simulink model "MMC_model"  (R2024b)
settings: Solver=ode23t  StartTime=0.0  StopTime=0.5  RelTol=1e-3
undefined symbols (not defined in the file): C0, f0, fs, L, Larm, Ldc, Rarm, Rdc, Ts
libraries: spsHalfBridgeMMCLib x36, spsSeriesRLCBranchLib x10, eePwmGeneratorMultilevel x6, spsDCVoltageSourceLib x2, spsGroundLib x1, spsThreePhaseSeriesRLCLoadLib x1, spsThreePhaseVIMeasurementLib x1, sps_lib x1
settings Model: Creator=nana  LastModifiedBy=nana

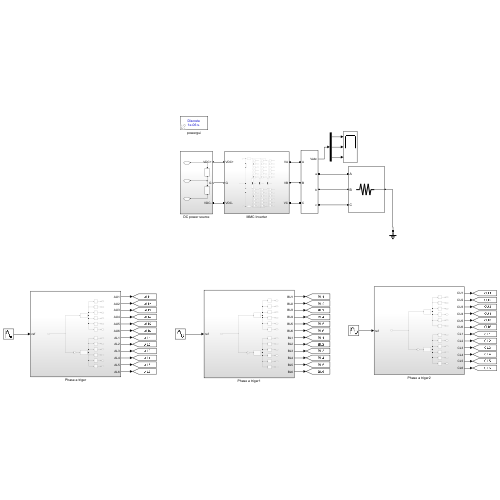
[thumbnail: Simulink's stored preview of the top-level diagram]
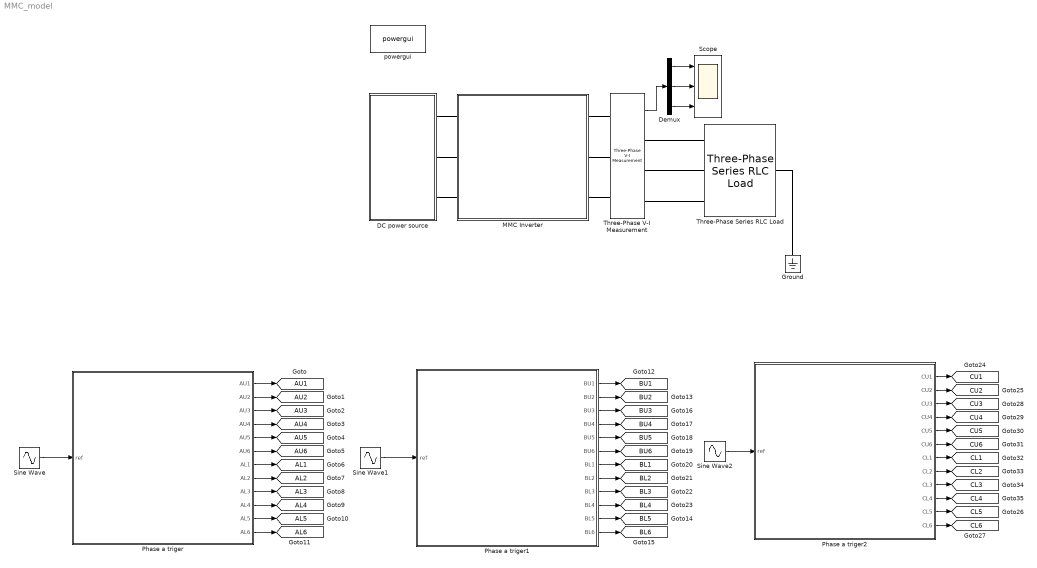
== system MMC_model ==
  DC power source : Subsystem
  Demux : Demux  Outputs=3
  Ground : spsGroundLib/Ground  LConnTagsString=a
  MMC Inverter : Subsystem
  Phase a triger : Subsystem
  Phase a triger1 : Subsystem
  Phase a triger2 : Subsystem
  Scope : Scope  NumInputPorts=3
  Sine Wave : Sin  Frequency=2*pi*f0  SampleTime=Ts
  Sine Wave1 : Sin  Frequency=2*pi*f0  Phase=-2*pi/3  SampleTime=Ts
  Sine Wave2 : Sin  Frequency=2*pi*f0  Phase=+2*pi/3  SampleTime=Ts
  Three-Phase Series RLC Load : spsThreePhaseSeriesRLCLoadLib/Three-Phase Series RLC Load  LConnTagsString=A|B|C  RConnTagsString=N  Configuration=Y (neutral)  NominalVoltage=12000  Vabc=[1e3 1e3 1e3]  Vabcp=[1e3 1e3 1e3]  NominalFrequency=50  UnbalancedPower=off  ActivePower=20e3  InductivePower=0  CapacitivePower=0  Pabc=[10e3 9e3 11e3]  QLabc=[100 90 110]  QCabc=[100 90 110]  Pabcp=[10e3 9e3 11e3]  QLabcp=[100 90 110]  QCabcp=[100 90 110]  Measurements=None  LoadType=constant Z
  Three-Phase V-I Measurement : spsThreePhaseVIMeasurementLib/Three-Phase V-I Measurement  VoltageMeasurement=phase-to-ground  SetLabelV=off  LabelV=Vabc  Vpu=off  VpuLL=off  CurrentMeasurement=yes  SetLabelI=on  LabelI=Iabc  Ipu=off  Pbase=100e6  Vbase=500e3  OutputType=Complex  PhasorSimulation=off  PSBequivalent=0
  powergui : sps_lib/powergui  Priority=1  SimulationMode=Discrete  SampleTime=1e-6  frequency=60  Iterations=50  frequencyindice=0  Pbase=100e6  ErrMax=1e-4  UnitsV=kV  UnitsW=MW  buscounter=0  FunctionMessages=off  echomessages=off  EnableUseOfTLC=off  CurrentSourceSwitches=off  DisableSnubberDevices=off  DisableRonSwitches=off  DisableVfSwitches=off  DisplayEquations=off  AutomaticDiscreteSolvers=off  SolverType=Tustin/Backward Euler (TBE)  Interpol=off  ExternalGateDelay=off  methode=off  Ts=100  x0status=blocks  SPID=on  SwTol=0  HookPort=off  NonlinearTolerance=1e-4  nMaxIteration=100  ContinueOnMaxIteration=off  RestoreLinks=warning  ResistiveCurrentMeasurement=off  Frange=[0:2:500]  Ylog=off  Xlog=on  ShowGrid=off  save=off  variable=ZData  structure=0  ZoomFFT=off  StartTime=0.0  cycles=1  DisplayStyle=1  fundamental=60  FreqAxis=off  MaxFrequency=1000  frequencyindicesteady=1  RmsSteady=1  display=off
  tag scope: AL1=global, AL2=global, AL3=global, AL4=global, AL5=global, AL6=global, AU1=global, AU2=global, AU3=global, AU4=global, AU5=global, AU6=global, BL1=global, BL2=global, BL3=global, BL4=global, BL5=global, BL6=global, BU1=global, BU2=global, BU3=global, BU4=global, BU5=global, BU6=global, CL1=global, CL2=global, CL3=global, CL4=global, CL5=global, CL6=global, CU1=global, CU2=global, CU3=global, CU4=global, CU5=global, CU6=global
  wires:
  Sine Wave/1 -> Phase a triger/1(ref)
  Sine Wave1/1 -> Phase a triger1/1(ref)
  Sine Wave2/1 -> Phase a triger2/1(ref)
  Phase a triger/1(AU1) -> [AU1]
  Phase a triger/2(AU2) -> [AU2]
  Phase a triger/12(AL6) -> [AL6]
  Phase a triger/11(AL5) -> [AL5]
  Phase a triger/10(AL4) -> [AL4]
  Phase a triger/9(AL3) -> [AL3]
  Phase a triger/8(AL2) -> [AL2]
  Phase a triger/7(AL1) -> [AL1]
  Phase a triger/6(AU6) -> [AU6]
  Phase a triger/5(AU5) -> [AU5]
  Phase a triger/4(AU4) -> [AU4]
  Phase a triger/3(AU3) -> [AU3]
  Phase a triger1/1(BU1) -> [BU1]
  Three-Phase V-I Measurement/1 -> Demux/1
  Demux/1 -> Scope/1
  Demux/2 -> Scope/2
  Demux/3 -> Scope/3
  Phase a triger1/2(BU2) -> [BU2]
  Phase a triger1/3(BU3) -> [BU3]
  Phase a triger1/4(BU4) -> [BU4]
  Phase a triger1/5(BU5) -> [BU5]
  Phase a triger1/6(BU6) -> [BU6]
  Phase a triger1/7(BL1) -> [BL1]
  Phase a triger1/8(BL2) -> [BL2]
  Phase a triger1/9(BL3) -> [BL3]
  Phase a triger1/10(BL4) -> [BL4]
  Phase a triger1/11(BL5) -> [BL5]
  Phase a triger1/12(BL6) -> [BL6]
  Phase a triger2/1(CU1) -> [CU1]
  Phase a triger2/2(CU2) -> [CU2]
  Phase a triger2/3(CU3) -> [CU3]
  Phase a triger2/4(CU4) -> [CU4]
  Phase a triger2/5(CU5) -> [CU5]
  Phase a triger2/6(CU6) -> [CU6]
  Phase a triger2/7(CL1) -> [CL1]
  Phase a triger2/8(CL2) -> [CL2]
  Phase a triger2/9(CL3) -> [CL3]
  Phase a triger2/10(CL4) -> [CL4]
  Phase a triger2/11(CL5) -> [CL5]
  Phase a triger2/12(CL6) -> [CL6]
  connections:
  DC power source/RConn1 -- MMC Inverter/LConn1
  Three-Phase Series RLC Load/RConn1 -- Ground/LConn1
  Three-Phase V-I Measurement/LConn1 -- MMC Inverter/RConn1
  Three-Phase V-I Measurement/LConn2 -- MMC Inverter/RConn2
  Three-Phase V-I Measurement/LConn3 -- MMC Inverter/RConn3
  Three-Phase Series RLC Load/LConn1 -- Three-Phase V-I Measurement/RConn1
  Three-Phase Series RLC Load/LConn2 -- Three-Phase V-I Measurement/RConn2
  Three-Phase Series RLC Load/LConn3 -- Three-Phase V-I Measurement/RConn3
  DC power source/RConn2 -- MMC Inverter/LConn2
  DC power source/RConn3 -- MMC Inverter/LConn3

== system MMC_model/DC power source ==
  DC Voltage Source : spsDCVoltageSourceLib/DC Voltage Source  Amplitude=6000  Measurements=None
  DC Voltage Source1 : spsDCVoltageSourceLib/DC Voltage Source  Amplitude=6000  Measurements=None
  VDC+ : PMIOPort  Side=Right
  G : PMIOPort  Port=2  Side=Right
  VDC- : PMIOPort  Port=3  Side=Right
  connections:
  DC Voltage Source/RConn1 -- VDC+/RConn1
  DC Voltage Source1/RConn1 -- G/RConn1 -- DC Voltage Source/LConn1
  VDC-/RConn1 -- DC Voltage Source1/LConn1

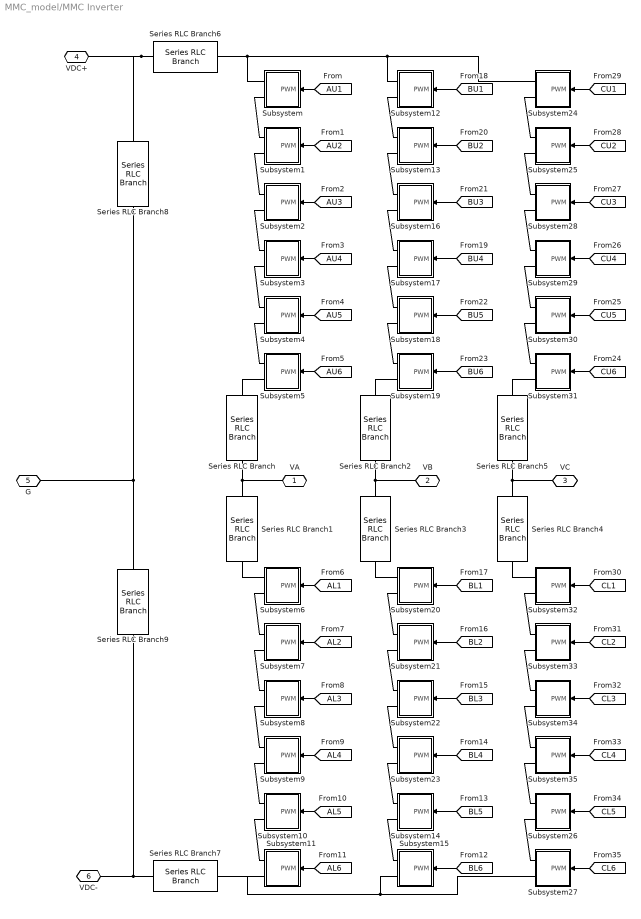
== system MMC_model/MMC Inverter ==
  Series RLC Branch{,1..5} (6 alike) : spsSeriesRLCBranchLib/Series RLC Branch  LConnTagsString=__new0  RConnTagsString=__new0  BranchType=RL  Resistance=Rarm  Inductance=Larm  SetiL0=off  InitialCurrent=0  Capacitance=1e-6  Setx0=off  InitialVoltage=0  Measurements=None
  Series RLC Branch6 : spsSeriesRLCBranchLib/Series RLC Branch  LConnTagsString=__new0  RConnTagsString=__new0  BranchType=RL  Resistance=Rdc  Inductance=Ldc  SetiL0=on  InitialCurrent=0  Capacitance=1e-6  Setx0=off  InitialVoltage=0  Measurements=None
  Series RLC Branch7 : spsSeriesRLCBranchLib/Series RLC Branch  LConnTagsString=__new0  RConnTagsString=__new0  BranchType=RL  Resistance=Rdc  Inductance=Ldc  SetiL0=on  InitialCurrent=0  Capacitance=1e-6  Setx0=off  InitialVoltage=0  Measurements=None
  Series RLC Branch8 : spsSeriesRLCBranchLib/Series RLC Branch  LConnTagsString=__new0  RConnTagsString=__new0  BranchType=RC  Resistance=1e-6  Inductance=L  SetiL0=on  InitialCurrent=0  Capacitance=8e-3  Setx0=on  InitialVoltage=3000  Measurements=None
  Series RLC Branch9 : spsSeriesRLCBranchLib/Series RLC Branch  LConnTagsString=__new0  RConnTagsString=__new0  BranchType=RC  Resistance=1e-6  Inductance=L  SetiL0=on  InitialCurrent=0  Capacitance=8e-3  Setx0=on  InitialVoltage=3000  Measurements=None
  Subsystem : Subsystem
  Subsystem1 : Subsystem
  Subsystem10 : Subsystem
  Subsystem11 : Subsystem
  Subsystem12 : Subsystem
  Subsystem13 : Subsystem
  Subsystem14 : Subsystem
  Subsystem15 : Subsystem
  Subsystem16 : Subsystem
  Subsystem17 : Subsystem
  Subsystem18 : Subsystem
  Subsystem19 : Subsystem
  Subsystem2 : Subsystem
  Subsystem20 : Subsystem
  Subsystem21 : Subsystem
  Subsystem22 : Subsystem
  Subsystem23 : Subsystem
  Subsystem24 : Subsystem
  Subsystem25 : Subsystem
  Subsystem26 : Subsystem
  Subsystem27 : Subsystem
  Subsystem28 : Subsystem
  Subsystem29 : Subsystem
  Subsystem3 : Subsystem
  Subsystem30 : Subsystem
  Subsystem31 : Subsystem
  Subsystem32 : Subsystem
  Subsystem33 : Subsystem
  Subsystem34 : Subsystem
  Subsystem35 : Subsystem
  Subsystem4 : Subsystem
  Subsystem5 : Subsystem
  Subsystem6 : Subsystem
  Subsystem7 : Subsystem
  Subsystem8 : Subsystem
  Subsystem9 : Subsystem
  VA : PMIOPort  Side=Right
  VB : PMIOPort  Port=2  Side=Right
  VC : PMIOPort  Port=3  Side=Right
  VDC+ : PMIOPort  Port=4  Side=Left
  G : PMIOPort  Port=5  Side=Left
  VDC- : PMIOPort  Port=6  Side=Left
  wires:
  [AL4] -> Subsystem9/1(PWM)
  [CL3] -> Subsystem34/1(PWM)
  [CU2] -> Subsystem25/1(PWM)
  [AL3] -> Subsystem8/1(PWM)
  [CL4] -> Subsystem35/1(PWM)
  [AL2] -> Subsystem7/1(PWM)
  [CU6] -> Subsystem31/1(PWM)
  [CL6] -> Subsystem27/1(PWM)
  [CL1] -> Subsystem32/1(PWM)
  [AL1] -> Subsystem6/1(PWM)
  [CL2] -> Subsystem33/1(PWM)
  [BU1] -> Subsystem12/1(PWM)
  [BU5] -> Subsystem18/1(PWM)
  [BL3] -> Subsystem22/1(PWM)
  [BU3] -> Subsystem16/1(PWM)
  [CU1] -> Subsystem24/1(PWM)
  [BL4] -> Subsystem23/1(PWM)
  [CU5] -> Subsystem30/1(PWM)
  [BL2] -> Subsystem21/1(PWM)
  [BU2] -> Subsystem13/1(PWM)
  [CU3] -> Subsystem28/1(PWM)
  [BL5] -> Subsystem14/1(PWM)
  [CL5] -> Subsystem26/1(PWM)
  [AU5] -> Subsystem4/1(PWM)
  [BL6] -> Subsystem15/1(PWM)
  [BU4] -> Subsystem17/1(PWM)
  [AU1] -> Subsystem/1(PWM)
  [AU6] -> Subsystem5/1(PWM)
  [AU3] -> Subsystem2/1(PWM)
  [AL5] -> Subsystem10/1(PWM)
  [AU2] -> Subsystem1/1(PWM)
  [BL1] -> Subsystem20/1(PWM)
  [CU4] -> Subsystem29/1(PWM)
  [AU4] -> Subsystem3/1(PWM)
  [BU6] -> Subsystem19/1(PWM)
  [AL6] -> Subsystem11/1(PWM)
  connections:
  Series RLC Branch6/RConn1 -- VDC+/RConn1 -- Series RLC Branch8/LConn1
  Subsystem3/RConn2 -- Subsystem4/RConn1
  Subsystem7/RConn2 -- Subsystem8/RConn1
  Subsystem29/RConn2 -- Subsystem30/RConn1
  Subsystem28/RConn2 -- Subsystem29/RConn1
  Subsystem12/RConn1 -- Series RLC Branch6/LConn1 -- Subsystem/RConn1 -- Subsystem24/RConn1
  Subsystem8/RConn2 -- Subsystem9/RConn1
  Series RLC Branch1/LConn1 -- VA/RConn1 -- Series RLC Branch/RConn1
  Series RLC Branch9/LConn1 -- G/RConn1 -- Series RLC Branch8/RConn1
  Subsystem/RConn2 -- Subsystem1/RConn1
  Subsystem30/RConn2 -- Subsystem31/RConn1
  Subsystem27/RConn2 -- Subsystem11/RConn2 -- Series RLC Branch7/LConn1 -- Subsystem15/RConn2
  Subsystem25/RConn2 -- Subsystem28/RConn1
  Subsystem4/RConn2 -- Subsystem5/RConn1
  Subsystem32/RConn2 -- Subsystem33/RConn1
  Subsystem24/RConn2 -- Subsystem25/RConn1
  Subsystem26/RConn2 -- Subsystem27/RConn1
  Subsystem17/RConn2 -- Subsystem18/RConn1
  Subsystem33/RConn2 -- Subsystem34/RConn1
  Series RLC Branch5/LConn1 -- Subsystem31/RConn2
  Subsystem21/RConn2 -- Subsystem22/RConn1
  Subsystem23/RConn2 -- Subsystem14/RConn1
  VC/RConn1 -- Series RLC Branch5/RConn1 -- Series RLC Branch4/LConn1
  Series RLC Branch9/RConn1 -- VDC-/RConn1 -- Series RLC Branch7/RConn1
  Subsystem34/RConn2 -- Subsystem35/RConn1
  Subsystem19/RConn2 -- Series RLC Branch2/LConn1
  Subsystem2/RConn2 -- Subsystem3/RConn1
  Subsystem35/RConn2 -- Subsystem26/RConn1
  Series RLC Branch4/RConn1 -- Subsystem32/RConn1
  Subsystem22/RConn2 -- Subsystem23/RConn1
  Series RLC Branch3/RConn1 -- Subsystem20/RConn1
  Subsystem6/RConn2 -- Subsystem7/RConn1
  Subsystem18/RConn2 -- Subsystem19/RConn1
  Subsystem1/RConn2 -- Subsystem2/RConn1
  Subsystem13/RConn2 -- Subsystem16/RConn1
  Subsystem5/RConn2 -- Series RLC Branch/LConn1
  Subsystem20/RConn2 -- Subsystem21/RConn1
  Subsystem10/RConn2 -- Subsystem11/RConn1
  Subsystem9/RConn2 -- Subsystem10/RConn1
  Series RLC Branch1/RConn1 -- Subsystem6/RConn1
  Subsystem14/RConn2 -- Subsystem15/RConn1
  Subsystem16/RConn2 -- Subsystem17/RConn1
  VB/RConn1 -- Series RLC Branch3/LConn1 -- Series RLC Branch2/RConn1
  Subsystem12/RConn2 -- Subsystem13/RConn1

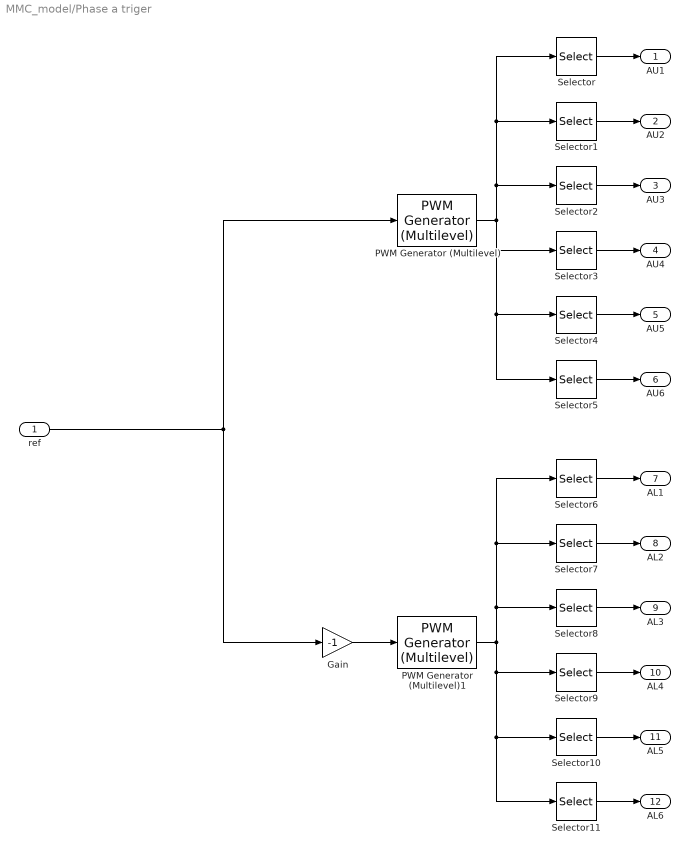
== system MMC_model/Phase a triger ==
  ref : Inport
  Gain : Gain  Gain=-1
  PWM Generator (Multilevel) : eePwmGeneratorMultilevel/PWM Generator (Multilevel)  topology=Half-bridge  Nsm=6  Tper=1/(2*fs)  Ts=Ts
      settings: LibrarySourceBlock=|
      | ee_sl_lib/Pulse Width
      | Modulation/PWM Generator
      | (Multilevel)
  PWM Generator (Multilevel)1 : eePwmGeneratorMultilevel/PWM Generator (Multilevel)  topology=Half-bridge  Nsm=6  Tper=1/(2*fs)  Ts=Ts
      settings: LibrarySourceBlock=|
      | ee_sl_lib/Pulse Width
      | Modulation/PWM Generator
      | (Multilevel)
  Selector : Selector  InputPortWidth=12  IndexOptions=Index vector (dialog)  Indices=[1:2]  OutputSizes=1
  Selector1 : Selector  InputPortWidth=12  IndexOptions=Index vector (dialog)  Indices=[3:4]  OutputSizes=1
  Selector10 : Selector  InputPortWidth=12  IndexOptions=Index vector (dialog)  Indices=[9:10]  OutputSizes=1
  Selector11 : Selector  InputPortWidth=12  IndexOptions=Index vector (dialog)  Indices=[11:12]  OutputSizes=1
  Selector2 : Selector  InputPortWidth=12  IndexOptions=Index vector (dialog)  Indices=[5:6]  OutputSizes=1
  Selector3 : Selector  InputPortWidth=12  IndexOptions=Index vector (dialog)  Indices=[7:8]  OutputSizes=1
  Selector4 : Selector  InputPortWidth=12  IndexOptions=Index vector (dialog)  Indices=[9:10]  OutputSizes=1
  Selector5 : Selector  InputPortWidth=12  IndexOptions=Index vector (dialog)  Indices=[11:12]  OutputSizes=1
  Selector6 : Selector  InputPortWidth=12  IndexOptions=Index vector (dialog)  Indices=[1:2]  OutputSizes=1
  Selector7 : Selector  InputPortWidth=12  IndexOptions=Index vector (dialog)  Indices=[3:4]  OutputSizes=1
  Selector8 : Selector  InputPortWidth=12  IndexOptions=Index vector (dialog)  Indices=[5:6]  OutputSizes=1
  Selector9 : Selector  InputPortWidth=12  IndexOptions=Index vector (dialog)  Indices=[7:8]  OutputSizes=1
  AU1 : Outport
  AU2 : Outport  Port=2
  AU3 : Outport  Port=3
  AU4 : Outport  Port=4
  AU5 : Outport  Port=5
  AU6 : Outport  Port=6
  AL1 : Outport  Port=7
  AL2 : Outport  Port=8
  AL3 : Outport  Port=9
  AL4 : Outport  Port=10
  AL5 : Outport  Port=11
  AL6 : Outport  Port=12
  wires:
  PWM Generator (Multilevel)1/1 -> Selector8/1, Selector7/1, Selector6/1, Selector9/1, Selector10/1, Selector11/1
  Selector3/1 -> AU4/1
  Selector2/1 -> AU3/1
  Selector4/1 -> AU5/1
  PWM Generator (Multilevel)/1 -> Selector2/1, Selector1/1, Selector/1, Selector3/1, Selector4/1, Selector5/1
  Selector6/1 -> AL1/1
  Selector7/1 -> AL2/1
  Selector1/1 -> AU2/1
  ref/1 -> PWM Generator (Multilevel)/1, Gain/1
  Selector11/1 -> AL6/1
  Selector5/1 -> AU6/1
  Gain/1 -> PWM Generator (Multilevel)1/1
  Selector8/1 -> AL3/1
  Selector/1 -> AU1/1
  Selector9/1 -> AL4/1
  Selector10/1 -> AL5/1

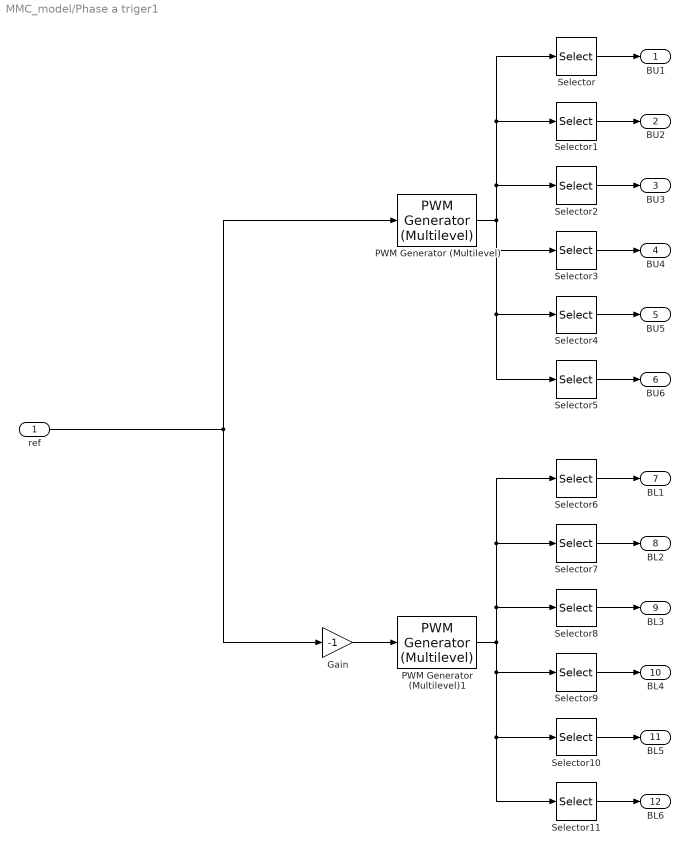
== system MMC_model/Phase a triger1 ==
  ref : Inport
  Gain : Gain  Gain=-1
  PWM Generator (Multilevel) : eePwmGeneratorMultilevel/PWM Generator (Multilevel)  topology=Half-bridge  Nsm=6  Tper=1/(2*fs)  Ts=Ts
  PWM Generator (Multilevel)1 : eePwmGeneratorMultilevel/PWM Generator (Multilevel)  topology=Half-bridge  Nsm=6  Tper=1/(2*fs)  Ts=Ts
  Selector : Selector  InputPortWidth=12  IndexOptions=Index vector (dialog)  Indices=[1:2]  OutputSizes=1
  Selector1 : Selector  InputPortWidth=12  IndexOptions=Index vector (dialog)  Indices=[3:4]  OutputSizes=1
  Selector10 : Selector  InputPortWidth=12  IndexOptions=Index vector (dialog)  Indices=[9:10]  OutputSizes=1
  Selector11 : Selector  InputPortWidth=12  IndexOptions=Index vector (dialog)  Indices=[11:12]  OutputSizes=1
  Selector2 : Selector  InputPortWidth=12  IndexOptions=Index vector (dialog)  Indices=[5:6]  OutputSizes=1
  Selector3 : Selector  InputPortWidth=12  IndexOptions=Index vector (dialog)  Indices=[7:8]  OutputSizes=1
  Selector4 : Selector  InputPortWidth=12  IndexOptions=Index vector (dialog)  Indices=[9:10]  OutputSizes=1
  Selector5 : Selector  InputPortWidth=12  IndexOptions=Index vector (dialog)  Indices=[11:12]  OutputSizes=1
  Selector6 : Selector  InputPortWidth=12  IndexOptions=Index vector (dialog)  Indices=[1:2]  OutputSizes=1
  Selector7 : Selector  InputPortWidth=12  IndexOptions=Index vector (dialog)  Indices=[3:4]  OutputSizes=1
  Selector8 : Selector  InputPortWidth=12  IndexOptions=Index vector (dialog)  Indices=[5:6]  OutputSizes=1
  Selector9 : Selector  InputPortWidth=12  IndexOptions=Index vector (dialog)  Indices=[7:8]  OutputSizes=1
  BU1 : Outport
  BU2 : Outport  Port=2
  BU3 : Outport  Port=3
  BU4 : Outport  Port=4
  BU5 : Outport  Port=5
  BU6 : Outport  Port=6
  BL1 : Outport  Port=7
  BL2 : Outport  Port=8
  BL3 : Outport  Port=9
  BL4 : Outport  Port=10
  BL5 : Outport  Port=11
  BL6 : Outport  Port=12
  wires:
  PWM Generator (Multilevel)1/1 -> Selector8/1, Selector7/1, Selector6/1, Selector9/1, Selector10/1, Selector11/1
  Selector3/1 -> BU4/1
  Selector2/1 -> BU3/1
  Selector4/1 -> BU5/1
  PWM Generator (Multilevel)/1 -> Selector2/1, Selector1/1, Selector/1, Selector3/1, Selector4/1, Selector5/1
  Selector6/1 -> BL1/1
  Selector7/1 -> BL2/1
  Selector1/1 -> BU2/1
  ref/1 -> PWM Generator (Multilevel)/1, Gain/1
  Selector11/1 -> BL6/1
  Selector5/1 -> BU6/1
  Gain/1 -> PWM Generator (Multilevel)1/1
  Selector8/1 -> BL3/1
  Selector/1 -> BU1/1
  Selector9/1 -> BL4/1
  Selector10/1 -> BL5/1

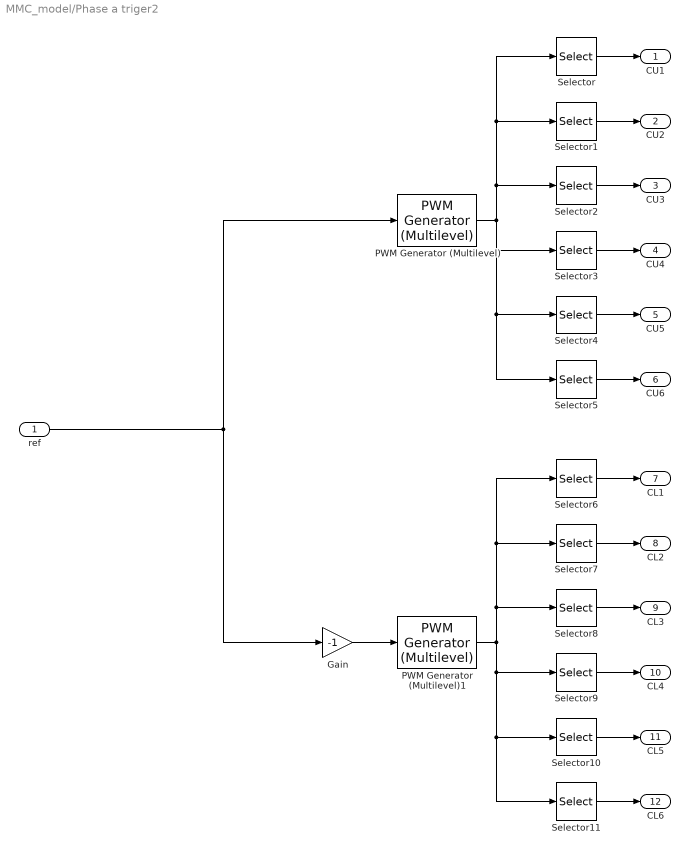
== system MMC_model/Phase a triger2 ==
  ref : Inport
  Gain : Gain  Gain=-1
  PWM Generator (Multilevel) : eePwmGeneratorMultilevel/PWM Generator (Multilevel)  topology=Half-bridge  Nsm=6  Tper=1/(2*fs)  Ts=Ts
  PWM Generator (Multilevel)1 : eePwmGeneratorMultilevel/PWM Generator (Multilevel)  topology=Half-bridge  Nsm=6  Tper=1/(2*fs)  Ts=Ts
  Selector : Selector  InputPortWidth=12  IndexOptions=Index vector (dialog)  Indices=[1:2]  OutputSizes=1
  Selector1 : Selector  InputPortWidth=12  IndexOptions=Index vector (dialog)  Indices=[3:4]  OutputSizes=1
  Selector10 : Selector  InputPortWidth=12  IndexOptions=Index vector (dialog)  Indices=[9:10]  OutputSizes=1
  Selector11 : Selector  InputPortWidth=12  IndexOptions=Index vector (dialog)  Indices=[11:12]  OutputSizes=1
  Selector2 : Selector  InputPortWidth=12  IndexOptions=Index vector (dialog)  Indices=[5:6]  OutputSizes=1
  Selector3 : Selector  InputPortWidth=12  IndexOptions=Index vector (dialog)  Indices=[7:8]  OutputSizes=1
  Selector4 : Selector  InputPortWidth=12  IndexOptions=Index vector (dialog)  Indices=[9:10]  OutputSizes=1
  Selector5 : Selector  InputPortWidth=12  IndexOptions=Index vector (dialog)  Indices=[11:12]  OutputSizes=1
  Selector6 : Selector  InputPortWidth=12  IndexOptions=Index vector (dialog)  Indices=[1:2]  OutputSizes=1
  Selector7 : Selector  InputPortWidth=12  IndexOptions=Index vector (dialog)  Indices=[3:4]  OutputSizes=1
  Selector8 : Selector  InputPortWidth=12  IndexOptions=Index vector (dialog)  Indices=[5:6]  OutputSizes=1
  Selector9 : Selector  InputPortWidth=12  IndexOptions=Index vector (dialog)  Indices=[7:8]  OutputSizes=1
  CU1 : Outport
  CU2 : Outport  Port=2
  CU3 : Outport  Port=3
  CU4 : Outport  Port=4
  CU5 : Outport  Port=5
  CU6 : Outport  Port=6
  CL1 : Outport  Port=7
  CL2 : Outport  Port=8
  CL3 : Outport  Port=9
  CL4 : Outport  Port=10
  CL5 : Outport  Port=11
  CL6 : Outport  Port=12
  wires:
  PWM Generator (Multilevel)1/1 -> Selector8/1, Selector7/1, Selector6/1, Selector9/1, Selector10/1, Selector11/1
  Selector3/1 -> CU4/1
  Selector2/1 -> CU3/1
  Selector4/1 -> CU5/1
  PWM Generator (Multilevel)/1 -> Selector2/1, Selector1/1, Selector/1, Selector3/1, Selector4/1, Selector5/1
  Selector6/1 -> CL1/1
  Selector7/1 -> CL2/1
  Selector1/1 -> CU2/1
  ref/1 -> PWM Generator (Multilevel)/1, Gain/1
  Selector11/1 -> CL6/1
  Selector5/1 -> CU6/1
  Gain/1 -> PWM Generator (Multilevel)1/1
  Selector8/1 -> CL3/1
  Selector/1 -> CU1/1
  Selector9/1 -> CL4/1
  Selector10/1 -> CL5/1

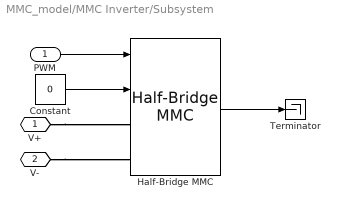
== system MMC_model/MMC Inverter/Subsystem ==
  PWM : Inport
  Constant : Constant  Value=0
  Half-Bridge MMC : spsHalfBridgeMMCLib/Half-Bridge MMC  ModelType=Switching devices  n=1  C=C0  Vc_Initial=V0  Ron=Ron  Rs=Rs  Cs=Cs  Ron_Diode=1e-3  Rs_Diode=1e6  Cs_Diode=inf  Vf_Diode=1e-3  Rs_CurrentSource=inf  Ts=10e-6
      settings: LibrarySourceBlock=sps_lib/Power Electronics/Half-Bridge MMC
  Terminator : Terminator
  V+ : PMIOPort  Side=Right
  V- : PMIOPort  Port=2  Side=Right
  wires:
  Half-Bridge MMC/1 -> Terminator/1
  Constant/1 -> Half-Bridge MMC/2
  PWM/1 -> Half-Bridge MMC/1
  connections:
  V-/RConn1 -- Half-Bridge MMC/LConn2
  V+/RConn1 -- Half-Bridge MMC/LConn1

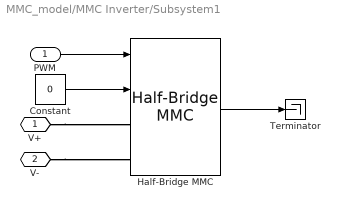
== system MMC_model/MMC Inverter/Subsystem1 ==
  PWM : Inport
  Constant : Constant  Value=0
  Half-Bridge MMC : spsHalfBridgeMMCLib/Half-Bridge MMC  ModelType=Switching devices  n=1  C=C0  Vc_Initial=V0  Ron=Ron  Rs=Rs  Cs=Cs  Ron_Diode=1e-3  Rs_Diode=1e6  Cs_Diode=inf  Vf_Diode=1e-3  Rs_CurrentSource=inf  Ts=10e-6
  Terminator : Terminator
  V+ : PMIOPort  Side=Right
  V- : PMIOPort  Port=2  Side=Right
  wires:
  Half-Bridge MMC/1 -> Terminator/1
  Constant/1 -> Half-Bridge MMC/2
  PWM/1 -> Half-Bridge MMC/1
  connections:
  V-/RConn1 -- Half-Bridge MMC/LConn2
  V+/RConn1 -- Half-Bridge MMC/LConn1

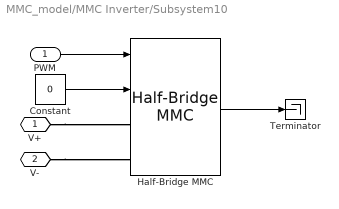
== system MMC_model/MMC Inverter/Subsystem10 ==
  PWM : Inport
  Constant : Constant  Value=0
  Half-Bridge MMC : spsHalfBridgeMMCLib/Half-Bridge MMC  ModelType=Switching devices  n=1  C=C0  Vc_Initial=V0  Ron=Ron  Rs=Rs  Cs=Cs  Ron_Diode=1e-3  Rs_Diode=1e6  Cs_Diode=inf  Vf_Diode=1e-3  Rs_CurrentSource=inf  Ts=10e-6
  Terminator : Terminator
  V+ : PMIOPort  Side=Right
  V- : PMIOPort  Port=2  Side=Right
  wires:
  Half-Bridge MMC/1 -> Terminator/1
  Constant/1 -> Half-Bridge MMC/2
  PWM/1 -> Half-Bridge MMC/1
  connections:
  V-/RConn1 -- Half-Bridge MMC/LConn2
  V+/RConn1 -- Half-Bridge MMC/LConn1

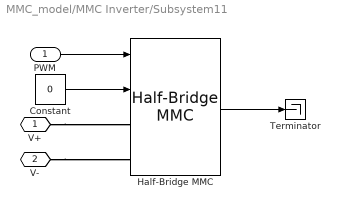
== system MMC_model/MMC Inverter/Subsystem11 ==
  PWM : Inport
  Constant : Constant  Value=0
  Half-Bridge MMC : spsHalfBridgeMMCLib/Half-Bridge MMC  ModelType=Switching devices  n=1  C=C0  Vc_Initial=V0  Ron=Ron  Rs=Rs  Cs=Cs  Ron_Diode=1e-3  Rs_Diode=1e6  Cs_Diode=inf  Vf_Diode=1e-3  Rs_CurrentSource=inf  Ts=10e-6
  Terminator : Terminator
  V+ : PMIOPort  Side=Right
  V- : PMIOPort  Port=2  Side=Right
  wires:
  Half-Bridge MMC/1 -> Terminator/1
  Constant/1 -> Half-Bridge MMC/2
  PWM/1 -> Half-Bridge MMC/1
  connections:
  V-/RConn1 -- Half-Bridge MMC/LConn2
  V+/RConn1 -- Half-Bridge MMC/LConn1

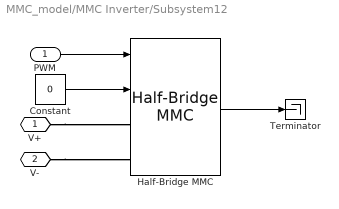
== system MMC_model/MMC Inverter/Subsystem12 ==
  PWM : Inport
  Constant : Constant  Value=0
  Half-Bridge MMC : spsHalfBridgeMMCLib/Half-Bridge MMC  ModelType=Switching devices  n=1  C=C0  Vc_Initial=V0  Ron=Ron  Rs=Rs  Cs=Cs  Ron_Diode=1e-3  Rs_Diode=1e6  Cs_Diode=inf  Vf_Diode=1e-3  Rs_CurrentSource=inf  Ts=10e-6
  Terminator : Terminator
  V+ : PMIOPort  Side=Right
  V- : PMIOPort  Port=2  Side=Right
  wires:
  Half-Bridge MMC/1 -> Terminator/1
  Constant/1 -> Half-Bridge MMC/2
  PWM/1 -> Half-Bridge MMC/1
  connections:
  V-/RConn1 -- Half-Bridge MMC/LConn2
  V+/RConn1 -- Half-Bridge MMC/LConn1

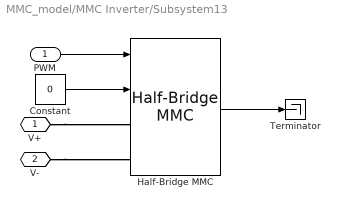
== system MMC_model/MMC Inverter/Subsystem13 ==
  PWM : Inport
  Constant : Constant  Value=0
  Half-Bridge MMC : spsHalfBridgeMMCLib/Half-Bridge MMC  ModelType=Switching devices  n=1  C=C0  Vc_Initial=V0  Ron=Ron  Rs=Rs  Cs=Cs  Ron_Diode=1e-3  Rs_Diode=1e6  Cs_Diode=inf  Vf_Diode=1e-3  Rs_CurrentSource=inf  Ts=10e-6
  Terminator : Terminator
  V+ : PMIOPort  Side=Right
  V- : PMIOPort  Port=2  Side=Right
  wires:
  Half-Bridge MMC/1 -> Terminator/1
  Constant/1 -> Half-Bridge MMC/2
  PWM/1 -> Half-Bridge MMC/1
  connections:
  V-/RConn1 -- Half-Bridge MMC/LConn2
  V+/RConn1 -- Half-Bridge MMC/LConn1

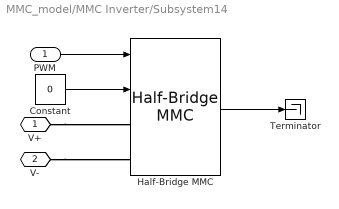
== system MMC_model/MMC Inverter/Subsystem14 ==
  PWM : Inport
  Constant : Constant  Value=0
  Half-Bridge MMC : spsHalfBridgeMMCLib/Half-Bridge MMC  ModelType=Switching devices  n=1  C=C0  Vc_Initial=V0  Ron=Ron  Rs=Rs  Cs=Cs  Ron_Diode=1e-3  Rs_Diode=1e6  Cs_Diode=inf  Vf_Diode=1e-3  Rs_CurrentSource=inf  Ts=10e-6
  Terminator : Terminator
  V+ : PMIOPort  Side=Right
  V- : PMIOPort  Port=2  Side=Right
  wires:
  Half-Bridge MMC/1 -> Terminator/1
  Constant/1 -> Half-Bridge MMC/2
  PWM/1 -> Half-Bridge MMC/1
  connections:
  V-/RConn1 -- Half-Bridge MMC/LConn2
  V+/RConn1 -- Half-Bridge MMC/LConn1

== system MMC_model/MMC Inverter/Subsystem15 ==
  PWM : Inport
  Constant : Constant  Value=0
  Half-Bridge MMC : spsHalfBridgeMMCLib/Half-Bridge MMC  ModelType=Switching devices  n=1  C=C0  Vc_Initial=V0  Ron=Ron  Rs=Rs  Cs=Cs  Ron_Diode=1e-3  Rs_Diode=1e6  Cs_Diode=inf  Vf_Diode=1e-3  Rs_CurrentSource=inf  Ts=10e-6
  Terminator : Terminator
  V+ : PMIOPort  Side=Right
  V- : PMIOPort  Port=2  Side=Right
  wires:
  Half-Bridge MMC/1 -> Terminator/1
  Constant/1 -> Half-Bridge MMC/2
  PWM/1 -> Half-Bridge MMC/1
  connections:
  V-/RConn1 -- Half-Bridge MMC/LConn2
  V+/RConn1 -- Half-Bridge MMC/LConn1

== system MMC_model/MMC Inverter/Subsystem16 ==
  PWM : Inport
  Constant : Constant  Value=0
  Half-Bridge MMC : spsHalfBridgeMMCLib/Half-Bridge MMC  ModelType=Switching devices  n=1  C=C0  Vc_Initial=V0  Ron=Ron  Rs=Rs  Cs=Cs  Ron_Diode=1e-3  Rs_Diode=1e6  Cs_Diode=inf  Vf_Diode=1e-3  Rs_CurrentSource=inf  Ts=10e-6
  Terminator : Terminator
  V+ : PMIOPort  Side=Right
  V- : PMIOPort  Port=2  Side=Right
  wires:
  Half-Bridge MMC/1 -> Terminator/1
  Constant/1 -> Half-Bridge MMC/2
  PWM/1 -> Half-Bridge MMC/1
  connections:
  V-/RConn1 -- Half-Bridge MMC/LConn2
  V+/RConn1 -- Half-Bridge MMC/LConn1

== system MMC_model/MMC Inverter/Subsystem17 ==
  PWM : Inport
  Constant : Constant  Value=0
  Half-Bridge MMC : spsHalfBridgeMMCLib/Half-Bridge MMC  ModelType=Switching devices  n=1  C=C0  Vc_Initial=V0  Ron=Ron  Rs=Rs  Cs=Cs  Ron_Diode=1e-3  Rs_Diode=1e6  Cs_Diode=inf  Vf_Diode=1e-3  Rs_CurrentSource=inf  Ts=10e-6
  Terminator : Terminator
  V+ : PMIOPort  Side=Right
  V- : PMIOPort  Port=2  Side=Right
  wires:
  Half-Bridge MMC/1 -> Terminator/1
  Constant/1 -> Half-Bridge MMC/2
  PWM/1 -> Half-Bridge MMC/1
  connections:
  V-/RConn1 -- Half-Bridge MMC/LConn2
  V+/RConn1 -- Half-Bridge MMC/LConn1

== system MMC_model/MMC Inverter/Subsystem18 ==
  PWM : Inport
  Constant : Constant  Value=0
  Half-Bridge MMC : spsHalfBridgeMMCLib/Half-Bridge MMC  ModelType=Switching devices  n=1  C=C0  Vc_Initial=V0  Ron=Ron  Rs=Rs  Cs=Cs  Ron_Diode=1e-3  Rs_Diode=1e6  Cs_Diode=inf  Vf_Diode=1e-3  Rs_CurrentSource=inf  Ts=10e-6
  Terminator : Terminator
  V+ : PMIOPort  Side=Right
  V- : PMIOPort  Port=2  Side=Right
  wires:
  Half-Bridge MMC/1 -> Terminator/1
  Constant/1 -> Half-Bridge MMC/2
  PWM/1 -> Half-Bridge MMC/1
  connections:
  V-/RConn1 -- Half-Bridge MMC/LConn2
  V+/RConn1 -- Half-Bridge MMC/LConn1

== system MMC_model/MMC Inverter/Subsystem19 ==
  PWM : Inport
  Constant : Constant  Value=0
  Half-Bridge MMC : spsHalfBridgeMMCLib/Half-Bridge MMC  ModelType=Switching devices  n=1  C=C0  Vc_Initial=V0  Ron=Ron  Rs=Rs  Cs=Cs  Ron_Diode=1e-3  Rs_Diode=1e6  Cs_Diode=inf  Vf_Diode=1e-3  Rs_CurrentSource=inf  Ts=10e-6
  Terminator : Terminator
  V+ : PMIOPort  Side=Right
  V- : PMIOPort  Port=2  Side=Right
  wires:
  Half-Bridge MMC/1 -> Terminator/1
  Constant/1 -> Half-Bridge MMC/2
  PWM/1 -> Half-Bridge MMC/1
  connections:
  V-/RConn1 -- Half-Bridge MMC/LConn2
  V+/RConn1 -- Half-Bridge MMC/LConn1

== system MMC_model/MMC Inverter/Subsystem2 ==
  PWM : Inport
  Constant : Constant  Value=0
  Half-Bridge MMC : spsHalfBridgeMMCLib/Half-Bridge MMC  ModelType=Switching devices  n=1  C=C0  Vc_Initial=V0  Ron=Ron  Rs=Rs  Cs=Cs  Ron_Diode=1e-3  Rs_Diode=1e6  Cs_Diode=inf  Vf_Diode=1e-3  Rs_CurrentSource=inf  Ts=10e-6
  Terminator : Terminator
  V+ : PMIOPort  Side=Right
  V- : PMIOPort  Port=2  Side=Right
  wires:
  Half-Bridge MMC/1 -> Terminator/1
  Constant/1 -> Half-Bridge MMC/2
  PWM/1 -> Half-Bridge MMC/1
  connections:
  V-/RConn1 -- Half-Bridge MMC/LConn2
  V+/RConn1 -- Half-Bridge MMC/LConn1

== system MMC_model/MMC Inverter/Subsystem20 ==
  PWM : Inport
  Constant : Constant  Value=0
  Half-Bridge MMC : spsHalfBridgeMMCLib/Half-Bridge MMC  ModelType=Switching devices  n=1  C=C0  Vc_Initial=V0  Ron=Ron  Rs=Rs  Cs=Cs  Ron_Diode=1e-3  Rs_Diode=1e6  Cs_Diode=inf  Vf_Diode=1e-3  Rs_CurrentSource=inf  Ts=10e-6
  Terminator : Terminator
  V+ : PMIOPort  Side=Right
  V- : PMIOPort  Port=2  Side=Right
  wires:
  Half-Bridge MMC/1 -> Terminator/1
  Constant/1 -> Half-Bridge MMC/2
  PWM/1 -> Half-Bridge MMC/1
  connections:
  V-/RConn1 -- Half-Bridge MMC/LConn2
  V+/RConn1 -- Half-Bridge MMC/LConn1

== system MMC_model/MMC Inverter/Subsystem21 ==
  PWM : Inport
  Constant : Constant  Value=0
  Half-Bridge MMC : spsHalfBridgeMMCLib/Half-Bridge MMC  ModelType=Switching devices  n=1  C=C0  Vc_Initial=V0  Ron=Ron  Rs=Rs  Cs=Cs  Ron_Diode=1e-3  Rs_Diode=1e6  Cs_Diode=inf  Vf_Diode=1e-3  Rs_CurrentSource=inf  Ts=10e-6
  Terminator : Terminator
  V+ : PMIOPort  Side=Right
  V- : PMIOPort  Port=2  Side=Right
  wires:
  Half-Bridge MMC/1 -> Terminator/1
  Constant/1 -> Half-Bridge MMC/2
  PWM/1 -> Half-Bridge MMC/1
  connections:
  V-/RConn1 -- Half-Bridge MMC/LConn2
  V+/RConn1 -- Half-Bridge MMC/LConn1

== system MMC_model/MMC Inverter/Subsystem22 ==
  PWM : Inport
  Constant : Constant  Value=0
  Half-Bridge MMC : spsHalfBridgeMMCLib/Half-Bridge MMC  ModelType=Switching devices  n=1  C=C0  Vc_Initial=V0  Ron=Ron  Rs=Rs  Cs=Cs  Ron_Diode=1e-3  Rs_Diode=1e6  Cs_Diode=inf  Vf_Diode=1e-3  Rs_CurrentSource=inf  Ts=10e-6
  Terminator : Terminator
  V+ : PMIOPort  Side=Right
  V- : PMIOPort  Port=2  Side=Right
  wires:
  Half-Bridge MMC/1 -> Terminator/1
  Constant/1 -> Half-Bridge MMC/2
  PWM/1 -> Half-Bridge MMC/1
  connections:
  V-/RConn1 -- Half-Bridge MMC/LConn2
  V+/RConn1 -- Half-Bridge MMC/LConn1

== system MMC_model/MMC Inverter/Subsystem23 ==
  PWM : Inport
  Constant : Constant  Value=0
  Half-Bridge MMC : spsHalfBridgeMMCLib/Half-Bridge MMC  ModelType=Switching devices  n=1  C=C0  Vc_Initial=V0  Ron=Ron  Rs=Rs  Cs=Cs  Ron_Diode=1e-3  Rs_Diode=1e6  Cs_Diode=inf  Vf_Diode=1e-3  Rs_CurrentSource=inf  Ts=10e-6
  Terminator : Terminator
  V+ : PMIOPort  Side=Right
  V- : PMIOPort  Port=2  Side=Right
  wires:
  Half-Bridge MMC/1 -> Terminator/1
  Constant/1 -> Half-Bridge MMC/2
  PWM/1 -> Half-Bridge MMC/1
  connections:
  V-/RConn1 -- Half-Bridge MMC/LConn2
  V+/RConn1 -- Half-Bridge MMC/LConn1

== system MMC_model/MMC Inverter/Subsystem24 ==
  PWM : Inport
  Constant : Constant  Value=0
  Half-Bridge MMC : spsHalfBridgeMMCLib/Half-Bridge MMC  ModelType=Switching devices  n=1  C=C0  Vc_Initial=V0  Ron=Ron  Rs=Rs  Cs=Cs  Ron_Diode=1e-3  Rs_Diode=1e6  Cs_Diode=inf  Vf_Diode=1e-3  Rs_CurrentSource=inf  Ts=10e-6
  Terminator : Terminator
  V+ : PMIOPort  Side=Right
  V- : PMIOPort  Port=2  Side=Right
  wires:
  Half-Bridge MMC/1 -> Terminator/1
  Constant/1 -> Half-Bridge MMC/2
  PWM/1 -> Half-Bridge MMC/1
  connections:
  V-/RConn1 -- Half-Bridge MMC/LConn2
  V+/RConn1 -- Half-Bridge MMC/LConn1

== system MMC_model/MMC Inverter/Subsystem25 ==
  PWM : Inport
  Constant : Constant  Value=0
  Half-Bridge MMC : spsHalfBridgeMMCLib/Half-Bridge MMC  ModelType=Switching devices  n=1  C=C0  Vc_Initial=V0  Ron=Ron  Rs=Rs  Cs=Cs  Ron_Diode=1e-3  Rs_Diode=1e6  Cs_Diode=inf  Vf_Diode=1e-3  Rs_CurrentSource=inf  Ts=10e-6
  Terminator : Terminator
  V+ : PMIOPort  Side=Right
  V- : PMIOPort  Port=2  Side=Right
  wires:
  Half-Bridge MMC/1 -> Terminator/1
  Constant/1 -> Half-Bridge MMC/2
  PWM/1 -> Half-Bridge MMC/1
  connections:
  V-/RConn1 -- Half-Bridge MMC/LConn2
  V+/RConn1 -- Half-Bridge MMC/LConn1

== system MMC_model/MMC Inverter/Subsystem26 ==
  PWM : Inport
  Constant : Constant  Value=0
  Half-Bridge MMC : spsHalfBridgeMMCLib/Half-Bridge MMC  ModelType=Switching devices  n=1  C=C0  Vc_Initial=V0  Ron=Ron  Rs=Rs  Cs=Cs  Ron_Diode=1e-3  Rs_Diode=1e6  Cs_Diode=inf  Vf_Diode=1e-3  Rs_CurrentSource=inf  Ts=10e-6
  Terminator : Terminator
  V+ : PMIOPort  Side=Right
  V- : PMIOPort  Port=2  Side=Right
  wires:
  Half-Bridge MMC/1 -> Terminator/1
  Constant/1 -> Half-Bridge MMC/2
  PWM/1 -> Half-Bridge MMC/1
  connections:
  V-/RConn1 -- Half-Bridge MMC/LConn2
  V+/RConn1 -- Half-Bridge MMC/LConn1

== system MMC_model/MMC Inverter/Subsystem27 ==
  PWM : Inport
  Constant : Constant  Value=0
  Half-Bridge MMC : spsHalfBridgeMMCLib/Half-Bridge MMC  ModelType=Switching devices  n=1  C=C0  Vc_Initial=V0  Ron=Ron  Rs=Rs  Cs=Cs  Ron_Diode=1e-3  Rs_Diode=1e6  Cs_Diode=inf  Vf_Diode=1e-3  Rs_CurrentSource=inf  Ts=10e-6
  Terminator : Terminator
  V+ : PMIOPort  Side=Right
  V- : PMIOPort  Port=2  Side=Right
  wires:
  Half-Bridge MMC/1 -> Terminator/1
  Constant/1 -> Half-Bridge MMC/2
  PWM/1 -> Half-Bridge MMC/1
  connections:
  V-/RConn1 -- Half-Bridge MMC/LConn2
  V+/RConn1 -- Half-Bridge MMC/LConn1

== system MMC_model/MMC Inverter/Subsystem28 ==
  PWM : Inport
  Constant : Constant  Value=0
  Half-Bridge MMC : spsHalfBridgeMMCLib/Half-Bridge MMC  ModelType=Switching devices  n=1  C=C0  Vc_Initial=V0  Ron=Ron  Rs=Rs  Cs=Cs  Ron_Diode=1e-3  Rs_Diode=1e6  Cs_Diode=inf  Vf_Diode=1e-3  Rs_CurrentSource=inf  Ts=10e-6
  Terminator : Terminator
  V+ : PMIOPort  Side=Right
  V- : PMIOPort  Port=2  Side=Right
  wires:
  Half-Bridge MMC/1 -> Terminator/1
  Constant/1 -> Half-Bridge MMC/2
  PWM/1 -> Half-Bridge MMC/1
  connections:
  V-/RConn1 -- Half-Bridge MMC/LConn2
  V+/RConn1 -- Half-Bridge MMC/LConn1

== system MMC_model/MMC Inverter/Subsystem29 ==
  PWM : Inport
  Constant : Constant  Value=0
  Half-Bridge MMC : spsHalfBridgeMMCLib/Half-Bridge MMC  ModelType=Switching devices  n=1  C=C0  Vc_Initial=V0  Ron=Ron  Rs=Rs  Cs=Cs  Ron_Diode=1e-3  Rs_Diode=1e6  Cs_Diode=inf  Vf_Diode=1e-3  Rs_CurrentSource=inf  Ts=10e-6
  Terminator : Terminator
  V+ : PMIOPort  Side=Right
  V- : PMIOPort  Port=2  Side=Right
  wires:
  Half-Bridge MMC/1 -> Terminator/1
  Constant/1 -> Half-Bridge MMC/2
  PWM/1 -> Half-Bridge MMC/1
  connections:
  V-/RConn1 -- Half-Bridge MMC/LConn2
  V+/RConn1 -- Half-Bridge MMC/LConn1

== system MMC_model/MMC Inverter/Subsystem3 ==
  PWM : Inport
  Constant : Constant  Value=0
  Half-Bridge MMC : spsHalfBridgeMMCLib/Half-Bridge MMC  ModelType=Switching devices  n=1  C=C0  Vc_Initial=V0  Ron=Ron  Rs=Rs  Cs=Cs  Ron_Diode=1e-3  Rs_Diode=1e6  Cs_Diode=inf  Vf_Diode=1e-3  Rs_CurrentSource=inf  Ts=10e-6
  Terminator : Terminator
  V+ : PMIOPort  Side=Right
  V- : PMIOPort  Port=2  Side=Right
  wires:
  Half-Bridge MMC/1 -> Terminator/1
  Constant/1 -> Half-Bridge MMC/2
  PWM/1 -> Half-Bridge MMC/1
  connections:
  V-/RConn1 -- Half-Bridge MMC/LConn2
  V+/RConn1 -- Half-Bridge MMC/LConn1

== system MMC_model/MMC Inverter/Subsystem30 ==
  PWM : Inport
  Constant : Constant  Value=0
  Half-Bridge MMC : spsHalfBridgeMMCLib/Half-Bridge MMC  ModelType=Switching devices  n=1  C=C0  Vc_Initial=V0  Ron=Ron  Rs=Rs  Cs=Cs  Ron_Diode=1e-3  Rs_Diode=1e6  Cs_Diode=inf  Vf_Diode=1e-3  Rs_CurrentSource=inf  Ts=10e-6
  Terminator : Terminator
  V+ : PMIOPort  Side=Right
  V- : PMIOPort  Port=2  Side=Right
  wires:
  Half-Bridge MMC/1 -> Terminator/1
  Constant/1 -> Half-Bridge MMC/2
  PWM/1 -> Half-Bridge MMC/1
  connections:
  V-/RConn1 -- Half-Bridge MMC/LConn2
  V+/RConn1 -- Half-Bridge MMC/LConn1

== system MMC_model/MMC Inverter/Subsystem31 ==
  PWM : Inport
  Constant : Constant  Value=0
  Half-Bridge MMC : spsHalfBridgeMMCLib/Half-Bridge MMC  ModelType=Switching devices  n=1  C=C0  Vc_Initial=V0  Ron=Ron  Rs=Rs  Cs=Cs  Ron_Diode=1e-3  Rs_Diode=1e6  Cs_Diode=inf  Vf_Diode=1e-3  Rs_CurrentSource=inf  Ts=10e-6
  Terminator : Terminator
  V+ : PMIOPort  Side=Right
  V- : PMIOPort  Port=2  Side=Right
  wires:
  Half-Bridge MMC/1 -> Terminator/1
  Constant/1 -> Half-Bridge MMC/2
  PWM/1 -> Half-Bridge MMC/1
  connections:
  V-/RConn1 -- Half-Bridge MMC/LConn2
  V+/RConn1 -- Half-Bridge MMC/LConn1

== system MMC_model/MMC Inverter/Subsystem32 ==
  PWM : Inport
  Constant : Constant  Value=0
  Half-Bridge MMC : spsHalfBridgeMMCLib/Half-Bridge MMC  ModelType=Switching devices  n=1  C=C0  Vc_Initial=V0  Ron=Ron  Rs=Rs  Cs=Cs  Ron_Diode=1e-3  Rs_Diode=1e6  Cs_Diode=inf  Vf_Diode=1e-3  Rs_CurrentSource=inf  Ts=10e-6
  Terminator : Terminator
  V+ : PMIOPort  Side=Right
  V- : PMIOPort  Port=2  Side=Right
  wires:
  Half-Bridge MMC/1 -> Terminator/1
  Constant/1 -> Half-Bridge MMC/2
  PWM/1 -> Half-Bridge MMC/1
  connections:
  V-/RConn1 -- Half-Bridge MMC/LConn2
  V+/RConn1 -- Half-Bridge MMC/LConn1

== system MMC_model/MMC Inverter/Subsystem33 ==
  PWM : Inport
  Constant : Constant  Value=0
  Half-Bridge MMC : spsHalfBridgeMMCLib/Half-Bridge MMC  ModelType=Switching devices  n=1  C=C0  Vc_Initial=V0  Ron=Ron  Rs=Rs  Cs=Cs  Ron_Diode=1e-3  Rs_Diode=1e6  Cs_Diode=inf  Vf_Diode=1e-3  Rs_CurrentSource=inf  Ts=10e-6
  Terminator : Terminator
  V+ : PMIOPort  Side=Right
  V- : PMIOPort  Port=2  Side=Right
  wires:
  Half-Bridge MMC/1 -> Terminator/1
  Constant/1 -> Half-Bridge MMC/2
  PWM/1 -> Half-Bridge MMC/1
  connections:
  V-/RConn1 -- Half-Bridge MMC/LConn2
  V+/RConn1 -- Half-Bridge MMC/LConn1

== system MMC_model/MMC Inverter/Subsystem34 ==
  PWM : Inport
  Constant : Constant  Value=0
  Half-Bridge MMC : spsHalfBridgeMMCLib/Half-Bridge MMC  ModelType=Switching devices  n=1  C=C0  Vc_Initial=V0  Ron=Ron  Rs=Rs  Cs=Cs  Ron_Diode=1e-3  Rs_Diode=1e6  Cs_Diode=inf  Vf_Diode=1e-3  Rs_CurrentSource=inf  Ts=10e-6
  Terminator : Terminator
  V+ : PMIOPort  Side=Right
  V- : PMIOPort  Port=2  Side=Right
  wires:
  Half-Bridge MMC/1 -> Terminator/1
  Constant/1 -> Half-Bridge MMC/2
  PWM/1 -> Half-Bridge MMC/1
  connections:
  V-/RConn1 -- Half-Bridge MMC/LConn2
  V+/RConn1 -- Half-Bridge MMC/LConn1

== system MMC_model/MMC Inverter/Subsystem35 ==
  PWM : Inport
  Constant : Constant  Value=0
  Half-Bridge MMC : spsHalfBridgeMMCLib/Half-Bridge MMC  ModelType=Switching devices  n=1  C=C0  Vc_Initial=V0  Ron=Ron  Rs=Rs  Cs=Cs  Ron_Diode=1e-3  Rs_Diode=1e6  Cs_Diode=inf  Vf_Diode=1e-3  Rs_CurrentSource=inf  Ts=10e-6
  Terminator : Terminator
  V+ : PMIOPort  Side=Right
  V- : PMIOPort  Port=2  Side=Right
  wires:
  Half-Bridge MMC/1 -> Terminator/1
  Constant/1 -> Half-Bridge MMC/2
  PWM/1 -> Half-Bridge MMC/1
  connections:
  V-/RConn1 -- Half-Bridge MMC/LConn2
  V+/RConn1 -- Half-Bridge MMC/LConn1

== system MMC_model/MMC Inverter/Subsystem4 ==
  PWM : Inport
  Constant : Constant  Value=0
  Half-Bridge MMC : spsHalfBridgeMMCLib/Half-Bridge MMC  ModelType=Switching devices  n=1  C=C0  Vc_Initial=V0  Ron=Ron  Rs=Rs  Cs=Cs  Ron_Diode=1e-3  Rs_Diode=1e6  Cs_Diode=inf  Vf_Diode=1e-3  Rs_CurrentSource=inf  Ts=10e-6
  Terminator : Terminator
  V+ : PMIOPort  Side=Right
  V- : PMIOPort  Port=2  Side=Right
  wires:
  Half-Bridge MMC/1 -> Terminator/1
  Constant/1 -> Half-Bridge MMC/2
  PWM/1 -> Half-Bridge MMC/1
  connections:
  V-/RConn1 -- Half-Bridge MMC/LConn2
  V+/RConn1 -- Half-Bridge MMC/LConn1

== system MMC_model/MMC Inverter/Subsystem5 ==
  PWM : Inport
  Constant : Constant  Value=0
  Half-Bridge MMC : spsHalfBridgeMMCLib/Half-Bridge MMC  ModelType=Switching devices  n=1  C=C0  Vc_Initial=V0  Ron=Ron  Rs=Rs  Cs=Cs  Ron_Diode=1e-3  Rs_Diode=1e6  Cs_Diode=inf  Vf_Diode=1e-3  Rs_CurrentSource=inf  Ts=10e-6
  Terminator : Terminator
  V+ : PMIOPort  Side=Right
  V- : PMIOPort  Port=2  Side=Right
  wires:
  Half-Bridge MMC/1 -> Terminator/1
  Constant/1 -> Half-Bridge MMC/2
  PWM/1 -> Half-Bridge MMC/1
  connections:
  V-/RConn1 -- Half-Bridge MMC/LConn2
  V+/RConn1 -- Half-Bridge MMC/LConn1

== system MMC_model/MMC Inverter/Subsystem6 ==
  PWM : Inport
  Constant : Constant  Value=0
  Half-Bridge MMC : spsHalfBridgeMMCLib/Half-Bridge MMC  ModelType=Switching devices  n=1  C=C0  Vc_Initial=V0  Ron=Ron  Rs=Rs  Cs=Cs  Ron_Diode=1e-3  Rs_Diode=1e6  Cs_Diode=inf  Vf_Diode=1e-3  Rs_CurrentSource=inf  Ts=10e-6
  Terminator : Terminator
  V+ : PMIOPort  Side=Right
  V- : PMIOPort  Port=2  Side=Right
  wires:
  Half-Bridge MMC/1 -> Terminator/1
  Constant/1 -> Half-Bridge MMC/2
  PWM/1 -> Half-Bridge MMC/1
  connections:
  V-/RConn1 -- Half-Bridge MMC/LConn2
  V+/RConn1 -- Half-Bridge MMC/LConn1

== system MMC_model/MMC Inverter/Subsystem7 ==
  PWM : Inport
  Constant : Constant  Value=0
  Half-Bridge MMC : spsHalfBridgeMMCLib/Half-Bridge MMC  ModelType=Switching devices  n=1  C=C0  Vc_Initial=V0  Ron=Ron  Rs=Rs  Cs=Cs  Ron_Diode=1e-3  Rs_Diode=1e6  Cs_Diode=inf  Vf_Diode=1e-3  Rs_CurrentSource=inf  Ts=10e-6
  Terminator : Terminator
  V+ : PMIOPort  Side=Right
  V- : PMIOPort  Port=2  Side=Right
  wires:
  Half-Bridge MMC/1 -> Terminator/1
  Constant/1 -> Half-Bridge MMC/2
  PWM/1 -> Half-Bridge MMC/1
  connections:
  V-/RConn1 -- Half-Bridge MMC/LConn2
  V+/RConn1 -- Half-Bridge MMC/LConn1

== system MMC_model/MMC Inverter/Subsystem8 ==
  PWM : Inport
  Constant : Constant  Value=0
  Half-Bridge MMC : spsHalfBridgeMMCLib/Half-Bridge MMC  ModelType=Switching devices  n=1  C=C0  Vc_Initial=V0  Ron=Ron  Rs=Rs  Cs=Cs  Ron_Diode=1e-3  Rs_Diode=1e6  Cs_Diode=inf  Vf_Diode=1e-3  Rs_CurrentSource=inf  Ts=10e-6
  Terminator : Terminator
  V+ : PMIOPort  Side=Right
  V- : PMIOPort  Port=2  Side=Right
  wires:
  Half-Bridge MMC/1 -> Terminator/1
  Constant/1 -> Half-Bridge MMC/2
  PWM/1 -> Half-Bridge MMC/1
  connections:
  V-/RConn1 -- Half-Bridge MMC/LConn2
  V+/RConn1 -- Half-Bridge MMC/LConn1

== system MMC_model/MMC Inverter/Subsystem9 ==
  PWM : Inport
  Constant : Constant  Value=0
  Half-Bridge MMC : spsHalfBridgeMMCLib/Half-Bridge MMC  ModelType=Switching devices  n=1  C=C0  Vc_Initial=V0  Ron=Ron  Rs=Rs  Cs=Cs  Ron_Diode=1e-3  Rs_Diode=1e6  Cs_Diode=inf  Vf_Diode=1e-3  Rs_CurrentSource=inf  Ts=10e-6
  Terminator : Terminator
  V+ : PMIOPort  Side=Right
  V- : PMIOPort  Port=2  Side=Right
  wires:
  Half-Bridge MMC/1 -> Terminator/1
  Constant/1 -> Half-Bridge MMC/2
  PWM/1 -> Half-Bridge MMC/1
  connections:
  V-/RConn1 -- Half-Bridge MMC/LConn2
  V+/RConn1 -- Half-Bridge MMC/LConn1
